simulink model "cos_sin_CORDIC"  (R2023b)
settings: Solver=FixedStepDiscrete  StartTime=0.0  StopTime=15*ts  RelTol=1e-3
undefined symbols (not defined in the file): ts
libraries: hdlsllib x30, simulink_extras x1
settings Model: DataTypeOverride=Off  Creator=adarwish  LastModifiedBy=hackathon_fpga
settings OptimizationCC: BlockReduction=off  ConditionallyExecuteInputs=off  DefaultParameterBehavior=Inlined  InheritOutputTypeSmallerThanSingle=on
settings DebuggingCC: AlgebraicLoopMsg=error  SingleTaskRateTransMsg=error  ParameterOverflowMsg=none  ParameterPrecisionLossMsg=none
settings HardwareCC: ProdBitPerPointer=32  ProdBitPerSizeT=32  ProdBitPerPtrDiffT=32  ProdLargestAtomicFloat=None  ProdIntDivRoundTo=Undefined  ProdEndianess=Unspecified  ProdWordSize=32  ProdHWDeviceType=ASIC/FPGA->ASIC/FPGA  TargetBitPerLong=64  TargetBitPerPointer=64  TargetBitPerSizeT=64  TargetBitPerPtrDiffT=64  TargetLongLongMode=on  TargetIntDivRoundTo=Zero  TargetEndianess=LittleEndian  TargetWordSize=64  TargetHWDeviceType=Custom Processor->MATLAB Host Computer  ProdEqTarget=off

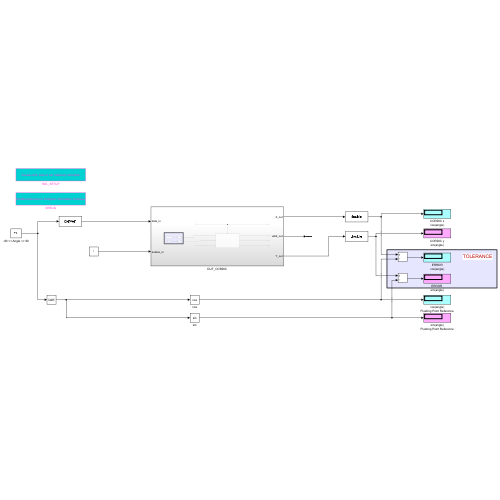
[thumbnail: Simulink's stored preview of the top-level diagram]
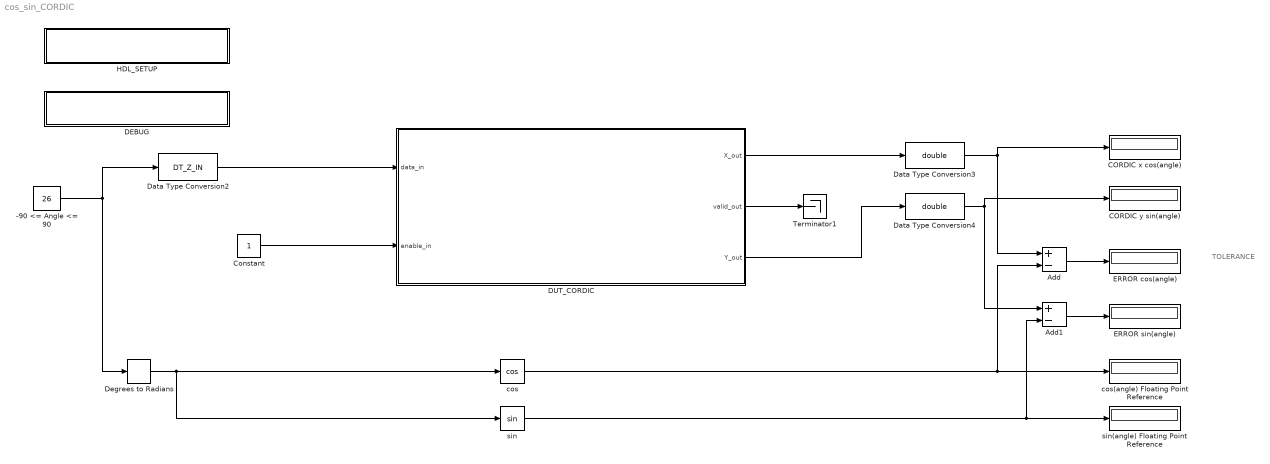
== system cos_sin_CORDIC ==
  note: TOLERANCE
  -90 <= Angle <= 90 : Constant  Value=26  SampleTime=ts
  Add : Sum  Inputs=+-
  Add1 : Sum  Inputs=+-
  CORDIC x cos(angle) : Display
  CORDIC y sin(angle) : Display
  Constant : Constant  OutDataTypeStr=boolean  SampleTime=-1
  DEBUG : Subsystem
      settings: OpenFcn=|
      | set_param(bdroot, 'ShowLineDimensions', 'on');
      | set_param(bdroot, 'SampleTimeColors', 'on');
      | set_param(bdroot, 'ShowLineDimensions', 'on');
      | disp('DONE Configuring Information Overlay')
      mask Display: disp(['Double-click here to configure Information Overlays'])
  DUT_CORDIC : Subsystem
  Data Type Conversion2 : DataTypeConversion  OutDataTypeStr=DT_Z_IN  RndMeth=Nearest  SampleTime=ts
  Data Type Conversion3 : DataTypeConversion  OutDataTypeStr=double  RndMeth=Nearest
  Data Type Conversion4 : DataTypeConversion  OutDataTypeStr=double  RndMeth=Nearest
  Degrees to Radians : simulink_extras/Transformations/Degrees to Radians
  ERROR cos(angle) : Display
  ERROR sin(angle) : Display
  HDL_SETUP : Subsystem
      settings: OpenFcn=hdlsetup(bdroot);
      mask Display: disp(['Double-click here to run hdlsetup command'])
  Terminator1 : Terminator
  cos : Trigonometry  Operator=cos
  cos(angle) Floating Point Reference : Display
  sin : Trigonometry
  sin(angle) Floating Point Reference : Display
  wires:
  sin/1 -> Add1/2, sin(angle) Floating Point Reference/1
  -90 <= Angle <= 90/1 -> Degrees to Radians/1, Data Type Conversion2/1
  Data Type Conversion4/1 -> CORDIC y sin(angle)/1, Add1/1
  Data Type Conversion3/1 -> CORDIC x cos(angle)/1, Add/1
  Add/1 -> ERROR cos(angle)/1
  Add1/1 -> ERROR sin(angle)/1
  Data Type Conversion2/1 -> DUT_CORDIC/1(data_in)
  cos/1 -> Add/2, cos(angle) Floating Point Reference/1
  Degrees to Radians/1 -> sin/1, cos/1
  Constant/1 -> DUT_CORDIC/2(enable_in)
  DUT_CORDIC/3(Y_out) -> Data Type Conversion4/1
  DUT_CORDIC/1(X_out) -> Data Type Conversion3/1
  DUT_CORDIC/2(valid_out) -> Terminator1/1

== system cos_sin_CORDIC/DEBUG ==

== system cos_sin_CORDIC/DUT_CORDIC ==
  note: PRE-SCALING
      | The input magnitude is prescaled to 1/1.6.
      | This means the finalmagnitude will be 1 and we do not need
      | to scale the output.
  data_in : Inport
  enable_in : Inport  Port=2
  1/Kn : Constant  Value=1/1.646743506596901  OutDataTypeStr=DT_X_IN  SampleTime=ts
  ALGORITHM : Subsystem
  Data Type Conversion : DataTypeConversion  OutDataTypeStr=DT_X_IN  RndMeth=Nearest  SampleTime=ts
  Data Type Conversion1 : DataTypeConversion  OutDataTypeStr=DT_Y_IN  RndMeth=Nearest  SampleTime=ts
  Set to 0 : Constant  Value=0  OutDataTypeStr=DT_Y_IN  SampleTime=ts
  Terminator : Terminator
  X_out : Outport
  valid_out : Outport  Port=2
  Y_out : Outport  Port=3
  wires:
  1/Kn/1 -> Data Type Conversion/1
  Set to 0/1 -> Data Type Conversion1/1
  Data Type Conversion/1 -> ALGORITHM/1(X In)
  Data Type Conversion1/1 -> ALGORITHM/2(Y In)
  data_in/1 -> ALGORITHM/3(Z In)
  ALGORITHM/3(Z Out) -> Terminator/1
  enable_in/1 -> ALGORITHM/Enable, valid_out/1
  ALGORITHM/1(X Out) -> X_out/1
  ALGORITHM/2(Y Out) -> Y_out/1

== system cos_sin_CORDIC/HDL_SETUP ==

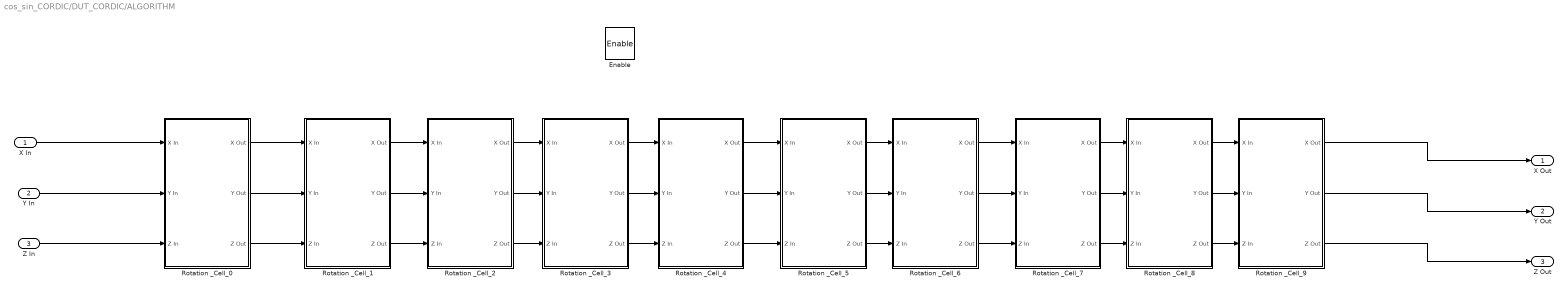
== system cos_sin_CORDIC/DUT_CORDIC/ALGORITHM ==
  X In : Inport
  Y In : Inport  Port=2
  Z In : Inport  Port=3
  Enable : EnablePort
  Rotation _Cell_0 : Subsystem  mask(Rotation Cell){i=0}
      mask prompts: i "Number of Iterations (i)"
  Rotation _Cell_1 : Subsystem  mask(Rotation Cell){i=1}
      mask prompts: i "Number of Iterations (i)"
  Rotation _Cell_2 : Subsystem  mask(Rotation Cell){i=2}
      mask prompts: i "Number of Iterations (i)"
  Rotation _Cell_3 : Subsystem  mask(Rotation Cell){i=3}
      mask prompts: i "Number of Iterations (i)"
  Rotation _Cell_4 : Subsystem  mask(Rotation Cell){i=4}
      mask prompts: i "Number of Iterations (i)"
  Rotation _Cell_5 : Subsystem  mask(Rotation Cell){i=5}
      mask prompts: i "Number of Iterations (i)"
  Rotation _Cell_6 : Subsystem  mask(Rotation Cell){i=6}
      mask prompts: i "Number of Iterations (i)"
  Rotation _Cell_7 : Subsystem  mask(Rotation Cell){i=7}
      mask prompts: i "Number of Iterations (i)"
  Rotation _Cell_8 : Subsystem  mask(Rotation Cell){i=8}
      mask prompts: i "Number of Iterations (i)"
  Rotation _Cell_9 : Subsystem  mask(Rotation Cell){i=9}
      mask prompts: i "Number of Iterations (i)"
  X Out : Outport  InitialOutput=0
  Y Out : Outport  Port=2  InitialOutput=0
  Z Out : Outport  Port=3  InitialOutput=0
  wires:
  Y In/1 -> Rotation _Cell_0/2(Y In)
  Rotation _Cell_0/2(Y Out) -> Rotation _Cell_1/2(Y In)
  Rotation _Cell_0/1(X Out) -> Rotation _Cell_1/1(X In)
  Rotation _Cell_0/3(Z Out) -> Rotation _Cell_1/3(Z In)
  X In/1 -> Rotation _Cell_0/1(X In)
  Z In/1 -> Rotation _Cell_0/3(Z In)
  Rotation _Cell_1/1(X Out) -> Rotation _Cell_2/1(X In)
  Rotation _Cell_1/2(Y Out) -> Rotation _Cell_2/2(Y In)
  Rotation _Cell_1/3(Z Out) -> Rotation _Cell_2/3(Z In)
  Rotation _Cell_2/1(X Out) -> Rotation _Cell_3/1(X In)
  Rotation _Cell_2/2(Y Out) -> Rotation _Cell_3/2(Y In)
  Rotation _Cell_2/3(Z Out) -> Rotation _Cell_3/3(Z In)
  Rotation _Cell_3/1(X Out) -> Rotation _Cell_4/1(X In)
  Rotation _Cell_3/2(Y Out) -> Rotation _Cell_4/2(Y In)
  Rotation _Cell_3/3(Z Out) -> Rotation _Cell_4/3(Z In)
  Rotation _Cell_4/1(X Out) -> Rotation _Cell_5/1(X In)
  Rotation _Cell_4/2(Y Out) -> Rotation _Cell_5/2(Y In)
  Rotation _Cell_4/3(Z Out) -> Rotation _Cell_5/3(Z In)
  Rotation _Cell_5/1(X Out) -> Rotation _Cell_6/1(X In)
  Rotation _Cell_5/2(Y Out) -> Rotation _Cell_6/2(Y In)
  Rotation _Cell_5/3(Z Out) -> Rotation _Cell_6/3(Z In)
  Rotation _Cell_6/1(X Out) -> Rotation _Cell_7/1(X In)
  Rotation _Cell_6/2(Y Out) -> Rotation _Cell_7/2(Y In)
  Rotation _Cell_6/3(Z Out) -> Rotation _Cell_7/3(Z In)
  Rotation _Cell_7/1(X Out) -> Rotation _Cell_8/1(X In)
  Rotation _Cell_7/2(Y Out) -> Rotation _Cell_8/2(Y In)
  Rotation _Cell_7/3(Z Out) -> Rotation _Cell_8/3(Z In)
  Rotation _Cell_8/1(X Out) -> Rotation _Cell_9/1(X In)
  Rotation _Cell_8/2(Y Out) -> Rotation _Cell_9/2(Y In)
  Rotation _Cell_8/3(Z Out) -> Rotation _Cell_9/3(Z In)
  Rotation _Cell_9/1(X Out) -> X Out/1
  Rotation _Cell_9/2(Y Out) -> Y Out/1
  Rotation _Cell_9/3(Z Out) -> Z Out/1

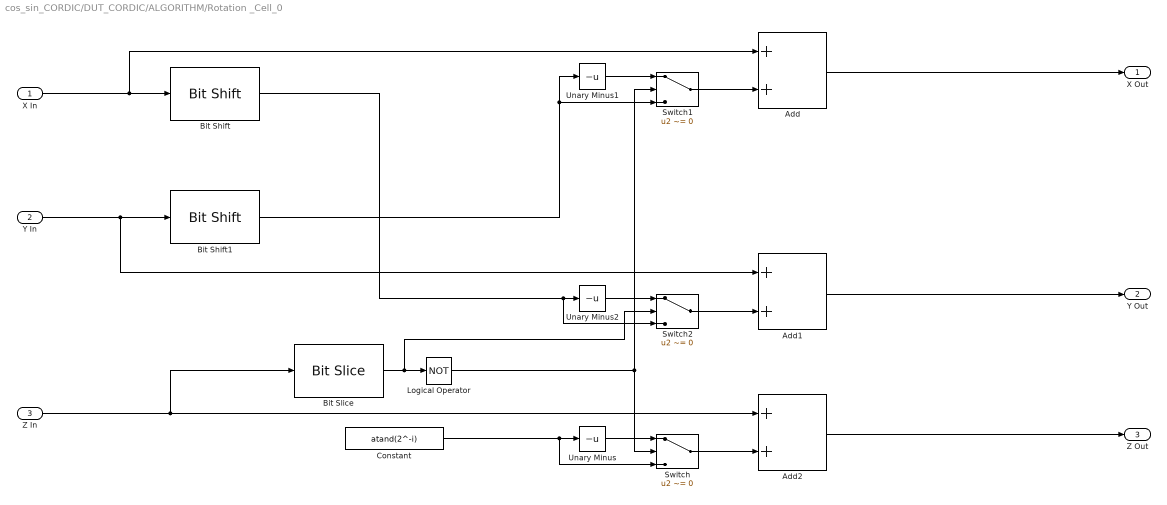
== system cos_sin_CORDIC/DUT_CORDIC/ALGORITHM/Rotation _Cell_0 ==
  X In : Inport
  Y In : Inport  Port=2
  Z In : Inport  Port=3
  Add : Sum  OutDataTypeStr=fixdt(1,15,12)
  Add1 : Sum  OutDataTypeStr=fixdt(1,15,12)
  Add2 : Sum  OutDataTypeStr=fixdt(1,20,12)
  Bit Shift : hdlsllib/Logic and Bit Operations/Bit Shift  mode=Shift Right Arithmetic  N=i
  Bit Shift1 : hdlsllib/Logic and Bit Operations/Bit Shift  mode=Shift Right Arithmetic  N=i
  Bit Slice : hdlsllib/Logic and Bit Operations/Bit Slice  lidx=19  ridx=19
  Constant : Constant  Value=atand(2^-i)  OutDataTypeStr=fixdt(1,20,12)  SampleTime=-1
  Logical Operator : Logic  Operator=NOT  AllPortsSameDT=off  OutDataTypeStr=boolean
  Switch : Switch  Criteria=u2 ~= 0  SaturateOnIntegerOverflow=off  InputSameDT=off
  Switch1 : Switch  Criteria=u2 ~= 0  SaturateOnIntegerOverflow=off  InputSameDT=off
  Switch2 : Switch  Criteria=u2 ~= 0  SaturateOnIntegerOverflow=off  InputSameDT=off
  Unary Minus : UnaryMinus
  Unary Minus1 : UnaryMinus
  Unary Minus2 : UnaryMinus
  X Out : Outport
  Y Out : Outport  Port=2
  Z Out : Outport  Port=3
  wires:
  Constant/1 -> Unary Minus/1, Switch/3
  Y In/1 -> Bit Shift1/1, Add1/1
  X In/1 -> Bit Shift/1, Add/1
  Add/1 -> X Out/1
  Unary Minus2/1 -> Switch2/1
  Unary Minus/1 -> Switch/1
  Add1/1 -> Y Out/1
  Switch1/1 -> Add/2
  Bit Shift/1 -> Switch2/3, Unary Minus2/1
  Switch2/1 -> Add1/2
  Unary Minus1/1 -> Switch1/1
  Bit Shift1/1 -> Switch1/3, Unary Minus1/1
  Z In/1 -> Bit Slice/1, Add2/1
  Bit Slice/1 -> Logical Operator/1, Switch2/2
  Switch/1 -> Add2/2
  Add2/1 -> Z Out/1
  Logical Operator/1 -> Switch/2, Switch1/2

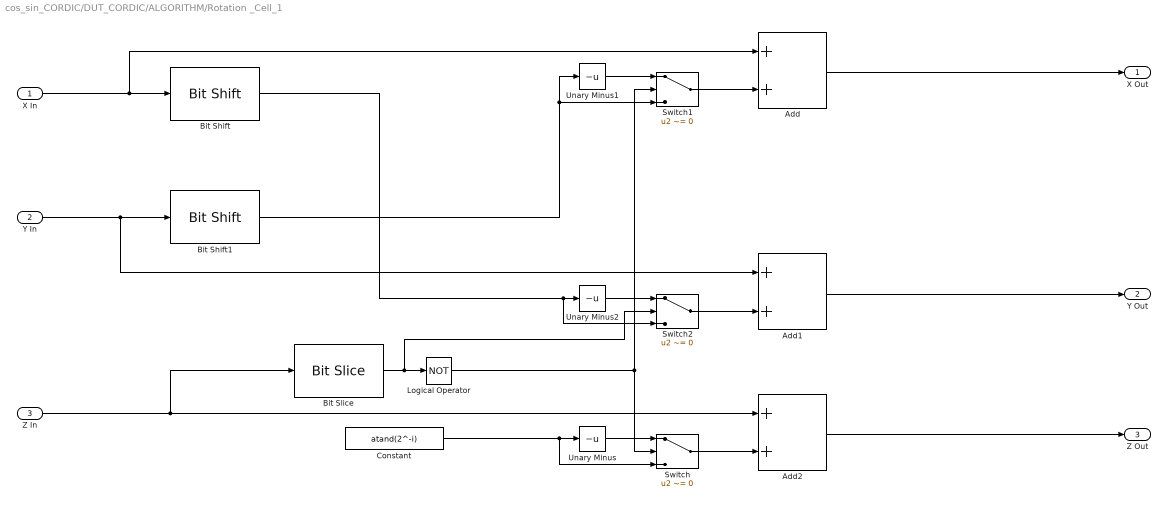
== system cos_sin_CORDIC/DUT_CORDIC/ALGORITHM/Rotation _Cell_1 ==
  X In : Inport
  Y In : Inport  Port=2
  Z In : Inport  Port=3
  Add : Sum  OutDataTypeStr=fixdt(1,15,12)
  Add1 : Sum  OutDataTypeStr=fixdt(1,15,12)
  Add2 : Sum  OutDataTypeStr=fixdt(1,20,12)
  Bit Shift : hdlsllib/Logic and Bit Operations/Bit Shift  mode=Shift Right Arithmetic  N=i
  Bit Shift1 : hdlsllib/Logic and Bit Operations/Bit Shift  mode=Shift Right Arithmetic  N=i
  Bit Slice : hdlsllib/Logic and Bit Operations/Bit Slice  lidx=19  ridx=19
  Constant : Constant  Value=atand(2^-i)  OutDataTypeStr=fixdt(1,20,12)  SampleTime=-1
  Logical Operator : Logic  Operator=NOT  AllPortsSameDT=off  OutDataTypeStr=boolean
  Switch : Switch  Criteria=u2 ~= 0  SaturateOnIntegerOverflow=off  InputSameDT=off
  Switch1 : Switch  Criteria=u2 ~= 0  SaturateOnIntegerOverflow=off  InputSameDT=off
  Switch2 : Switch  Criteria=u2 ~= 0  SaturateOnIntegerOverflow=off  InputSameDT=off
  Unary Minus : UnaryMinus
  Unary Minus1 : UnaryMinus
  Unary Minus2 : UnaryMinus
  X Out : Outport
  Y Out : Outport  Port=2
  Z Out : Outport  Port=3
  wires:
  Constant/1 -> Unary Minus/1, Switch/3
  Y In/1 -> Bit Shift1/1, Add1/1
  X In/1 -> Bit Shift/1, Add/1
  Add/1 -> X Out/1
  Unary Minus2/1 -> Switch2/1
  Unary Minus/1 -> Switch/1
  Add1/1 -> Y Out/1
  Switch1/1 -> Add/2
  Bit Shift/1 -> Switch2/3, Unary Minus2/1
  Switch2/1 -> Add1/2
  Unary Minus1/1 -> Switch1/1
  Bit Shift1/1 -> Switch1/3, Unary Minus1/1
  Z In/1 -> Bit Slice/1, Add2/1
  Bit Slice/1 -> Logical Operator/1, Switch2/2
  Switch/1 -> Add2/2
  Add2/1 -> Z Out/1
  Logical Operator/1 -> Switch/2, Switch1/2

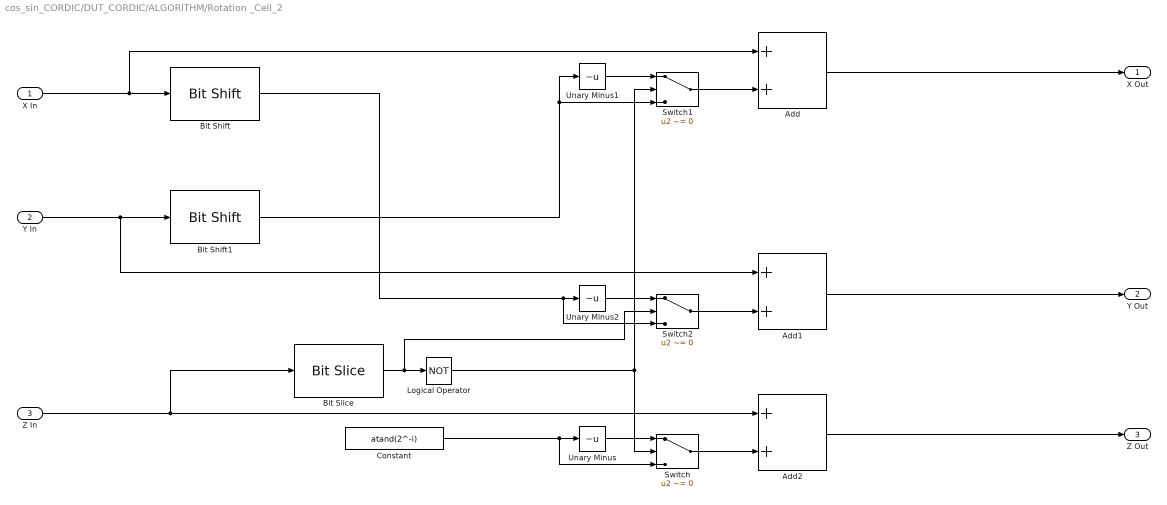
== system cos_sin_CORDIC/DUT_CORDIC/ALGORITHM/Rotation _Cell_2 ==
  X In : Inport
  Y In : Inport  Port=2
  Z In : Inport  Port=3
  Add : Sum  OutDataTypeStr=fixdt(1,15,12)
  Add1 : Sum  OutDataTypeStr=fixdt(1,15,12)
  Add2 : Sum  OutDataTypeStr=fixdt(1,20,12)
  Bit Shift : hdlsllib/Logic and Bit Operations/Bit Shift  mode=Shift Right Arithmetic  N=i
  Bit Shift1 : hdlsllib/Logic and Bit Operations/Bit Shift  mode=Shift Right Arithmetic  N=i
  Bit Slice : hdlsllib/Logic and Bit Operations/Bit Slice  lidx=19  ridx=19
  Constant : Constant  Value=atand(2^-i)  OutDataTypeStr=fixdt(1,20,12)  SampleTime=-1
  Logical Operator : Logic  Operator=NOT  AllPortsSameDT=off  OutDataTypeStr=boolean
  Switch : Switch  Criteria=u2 ~= 0  SaturateOnIntegerOverflow=off  InputSameDT=off
  Switch1 : Switch  Criteria=u2 ~= 0  SaturateOnIntegerOverflow=off  InputSameDT=off
  Switch2 : Switch  Criteria=u2 ~= 0  SaturateOnIntegerOverflow=off  InputSameDT=off
  Unary Minus : UnaryMinus
  Unary Minus1 : UnaryMinus
  Unary Minus2 : UnaryMinus
  X Out : Outport
  Y Out : Outport  Port=2
  Z Out : Outport  Port=3
  wires:
  Constant/1 -> Unary Minus/1, Switch/3
  Y In/1 -> Bit Shift1/1, Add1/1
  X In/1 -> Bit Shift/1, Add/1
  Add/1 -> X Out/1
  Unary Minus2/1 -> Switch2/1
  Unary Minus/1 -> Switch/1
  Add1/1 -> Y Out/1
  Switch1/1 -> Add/2
  Bit Shift/1 -> Switch2/3, Unary Minus2/1
  Switch2/1 -> Add1/2
  Unary Minus1/1 -> Switch1/1
  Bit Shift1/1 -> Switch1/3, Unary Minus1/1
  Z In/1 -> Bit Slice/1, Add2/1
  Bit Slice/1 -> Logical Operator/1, Switch2/2
  Switch/1 -> Add2/2
  Add2/1 -> Z Out/1
  Logical Operator/1 -> Switch/2, Switch1/2

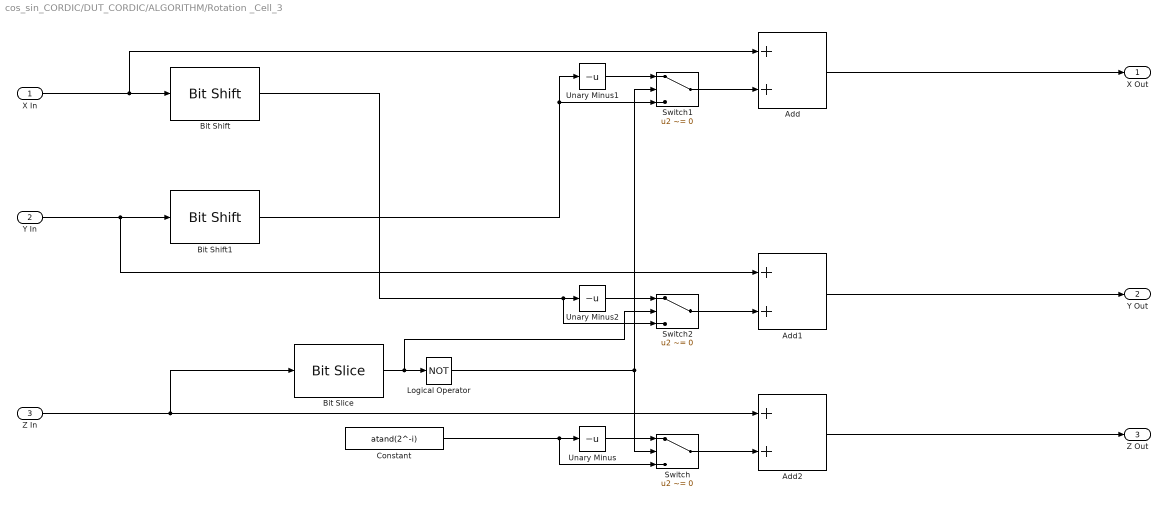
== system cos_sin_CORDIC/DUT_CORDIC/ALGORITHM/Rotation _Cell_3 ==
  X In : Inport
  Y In : Inport  Port=2
  Z In : Inport  Port=3
  Add : Sum  OutDataTypeStr=fixdt(1,15,12)
  Add1 : Sum  OutDataTypeStr=fixdt(1,15,12)
  Add2 : Sum  OutDataTypeStr=fixdt(1,20,12)
  Bit Shift : hdlsllib/Logic and Bit Operations/Bit Shift  mode=Shift Right Arithmetic  N=i
  Bit Shift1 : hdlsllib/Logic and Bit Operations/Bit Shift  mode=Shift Right Arithmetic  N=i
  Bit Slice : hdlsllib/Logic and Bit Operations/Bit Slice  lidx=19  ridx=19
  Constant : Constant  Value=atand(2^-i)  OutDataTypeStr=fixdt(1,20,12)  SampleTime=-1
  Logical Operator : Logic  Operator=NOT  AllPortsSameDT=off  OutDataTypeStr=boolean
  Switch : Switch  Criteria=u2 ~= 0  SaturateOnIntegerOverflow=off  InputSameDT=off
  Switch1 : Switch  Criteria=u2 ~= 0  SaturateOnIntegerOverflow=off  InputSameDT=off
  Switch2 : Switch  Criteria=u2 ~= 0  SaturateOnIntegerOverflow=off  InputSameDT=off
  Unary Minus : UnaryMinus
  Unary Minus1 : UnaryMinus
  Unary Minus2 : UnaryMinus
  X Out : Outport
  Y Out : Outport  Port=2
  Z Out : Outport  Port=3
  wires:
  Constant/1 -> Unary Minus/1, Switch/3
  Y In/1 -> Bit Shift1/1, Add1/1
  X In/1 -> Bit Shift/1, Add/1
  Add/1 -> X Out/1
  Unary Minus2/1 -> Switch2/1
  Unary Minus/1 -> Switch/1
  Add1/1 -> Y Out/1
  Switch1/1 -> Add/2
  Bit Shift/1 -> Switch2/3, Unary Minus2/1
  Switch2/1 -> Add1/2
  Unary Minus1/1 -> Switch1/1
  Bit Shift1/1 -> Switch1/3, Unary Minus1/1
  Z In/1 -> Bit Slice/1, Add2/1
  Bit Slice/1 -> Logical Operator/1, Switch2/2
  Switch/1 -> Add2/2
  Add2/1 -> Z Out/1
  Logical Operator/1 -> Switch/2, Switch1/2

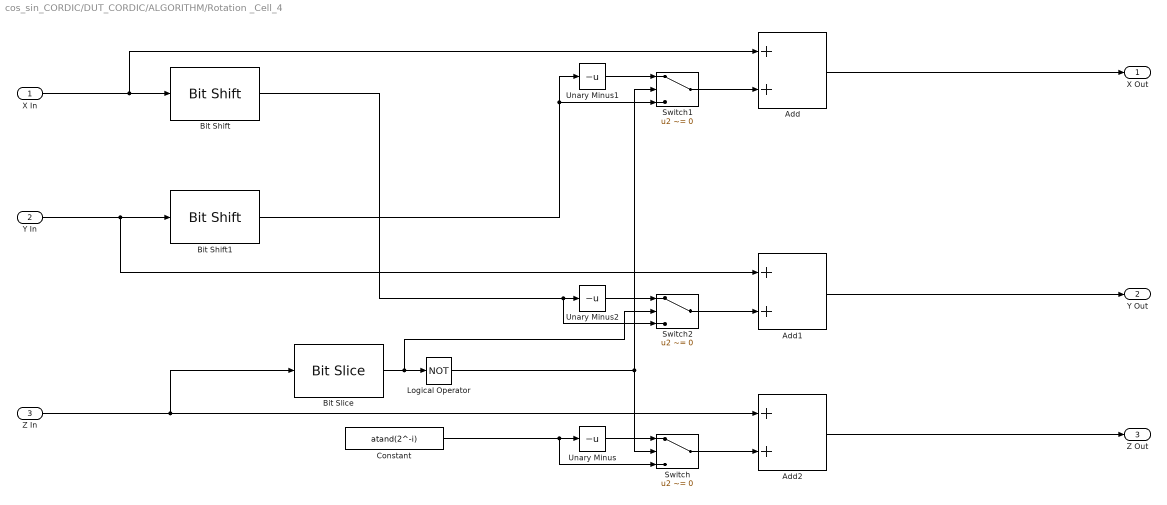
== system cos_sin_CORDIC/DUT_CORDIC/ALGORITHM/Rotation _Cell_4 ==
  X In : Inport
  Y In : Inport  Port=2
  Z In : Inport  Port=3
  Add : Sum  OutDataTypeStr=fixdt(1,15,12)
  Add1 : Sum  OutDataTypeStr=fixdt(1,15,12)
  Add2 : Sum  OutDataTypeStr=fixdt(1,20,12)
  Bit Shift : hdlsllib/Logic and Bit Operations/Bit Shift  mode=Shift Right Arithmetic  N=i
  Bit Shift1 : hdlsllib/Logic and Bit Operations/Bit Shift  mode=Shift Right Arithmetic  N=i
  Bit Slice : hdlsllib/Logic and Bit Operations/Bit Slice  lidx=19  ridx=19
  Constant : Constant  Value=atand(2^-i)  OutDataTypeStr=fixdt(1,20,12)  SampleTime=-1
  Logical Operator : Logic  Operator=NOT  AllPortsSameDT=off  OutDataTypeStr=boolean
  Switch : Switch  Criteria=u2 ~= 0  SaturateOnIntegerOverflow=off  InputSameDT=off
  Switch1 : Switch  Criteria=u2 ~= 0  SaturateOnIntegerOverflow=off  InputSameDT=off
  Switch2 : Switch  Criteria=u2 ~= 0  SaturateOnIntegerOverflow=off  InputSameDT=off
  Unary Minus : UnaryMinus
  Unary Minus1 : UnaryMinus
  Unary Minus2 : UnaryMinus
  X Out : Outport
  Y Out : Outport  Port=2
  Z Out : Outport  Port=3
  wires:
  Constant/1 -> Unary Minus/1, Switch/3
  Y In/1 -> Bit Shift1/1, Add1/1
  X In/1 -> Bit Shift/1, Add/1
  Add/1 -> X Out/1
  Unary Minus2/1 -> Switch2/1
  Unary Minus/1 -> Switch/1
  Add1/1 -> Y Out/1
  Switch1/1 -> Add/2
  Bit Shift/1 -> Switch2/3, Unary Minus2/1
  Switch2/1 -> Add1/2
  Unary Minus1/1 -> Switch1/1
  Bit Shift1/1 -> Switch1/3, Unary Minus1/1
  Z In/1 -> Bit Slice/1, Add2/1
  Bit Slice/1 -> Logical Operator/1, Switch2/2
  Switch/1 -> Add2/2
  Add2/1 -> Z Out/1
  Logical Operator/1 -> Switch/2, Switch1/2

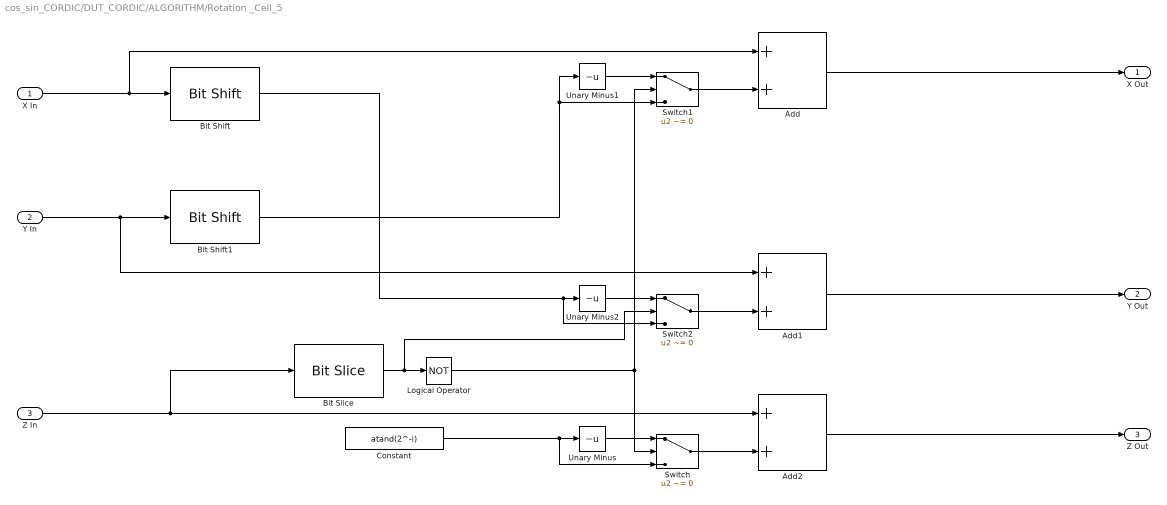
== system cos_sin_CORDIC/DUT_CORDIC/ALGORITHM/Rotation _Cell_5 ==
  X In : Inport
  Y In : Inport  Port=2
  Z In : Inport  Port=3
  Add : Sum  OutDataTypeStr=fixdt(1,15,12)
  Add1 : Sum  OutDataTypeStr=fixdt(1,15,12)
  Add2 : Sum  OutDataTypeStr=fixdt(1,20,12)
  Bit Shift : hdlsllib/Logic and Bit Operations/Bit Shift  mode=Shift Right Arithmetic  N=i
  Bit Shift1 : hdlsllib/Logic and Bit Operations/Bit Shift  mode=Shift Right Arithmetic  N=i
  Bit Slice : hdlsllib/Logic and Bit Operations/Bit Slice  lidx=19  ridx=19
  Constant : Constant  Value=atand(2^-i)  OutDataTypeStr=fixdt(1,20,12)  SampleTime=-1
  Logical Operator : Logic  Operator=NOT  AllPortsSameDT=off  OutDataTypeStr=boolean
  Switch : Switch  Criteria=u2 ~= 0  SaturateOnIntegerOverflow=off  InputSameDT=off
  Switch1 : Switch  Criteria=u2 ~= 0  SaturateOnIntegerOverflow=off  InputSameDT=off
  Switch2 : Switch  Criteria=u2 ~= 0  SaturateOnIntegerOverflow=off  InputSameDT=off
  Unary Minus : UnaryMinus
  Unary Minus1 : UnaryMinus
  Unary Minus2 : UnaryMinus
  X Out : Outport
  Y Out : Outport  Port=2
  Z Out : Outport  Port=3
  wires:
  Constant/1 -> Unary Minus/1, Switch/3
  Y In/1 -> Bit Shift1/1, Add1/1
  X In/1 -> Bit Shift/1, Add/1
  Add/1 -> X Out/1
  Unary Minus2/1 -> Switch2/1
  Unary Minus/1 -> Switch/1
  Add1/1 -> Y Out/1
  Switch1/1 -> Add/2
  Bit Shift/1 -> Switch2/3, Unary Minus2/1
  Switch2/1 -> Add1/2
  Unary Minus1/1 -> Switch1/1
  Bit Shift1/1 -> Switch1/3, Unary Minus1/1
  Z In/1 -> Bit Slice/1, Add2/1
  Bit Slice/1 -> Logical Operator/1, Switch2/2
  Switch/1 -> Add2/2
  Add2/1 -> Z Out/1
  Logical Operator/1 -> Switch/2, Switch1/2

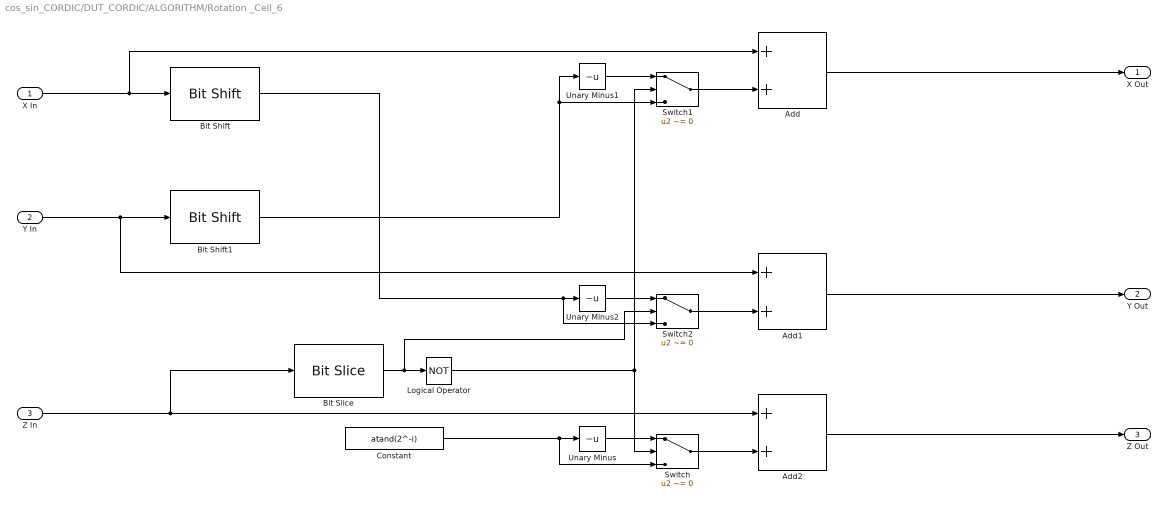
== system cos_sin_CORDIC/DUT_CORDIC/ALGORITHM/Rotation _Cell_6 ==
  X In : Inport
  Y In : Inport  Port=2
  Z In : Inport  Port=3
  Add : Sum  OutDataTypeStr=fixdt(1,15,12)
  Add1 : Sum  OutDataTypeStr=fixdt(1,15,12)
  Add2 : Sum  OutDataTypeStr=fixdt(1,20,12)
  Bit Shift : hdlsllib/Logic and Bit Operations/Bit Shift  mode=Shift Right Arithmetic  N=i
  Bit Shift1 : hdlsllib/Logic and Bit Operations/Bit Shift  mode=Shift Right Arithmetic  N=i
  Bit Slice : hdlsllib/Logic and Bit Operations/Bit Slice  lidx=19  ridx=19
  Constant : Constant  Value=atand(2^-i)  OutDataTypeStr=fixdt(1,20,12)  SampleTime=-1
  Logical Operator : Logic  Operator=NOT  AllPortsSameDT=off  OutDataTypeStr=boolean
  Switch : Switch  Criteria=u2 ~= 0  SaturateOnIntegerOverflow=off  InputSameDT=off
  Switch1 : Switch  Criteria=u2 ~= 0  SaturateOnIntegerOverflow=off  InputSameDT=off
  Switch2 : Switch  Criteria=u2 ~= 0  SaturateOnIntegerOverflow=off  InputSameDT=off
  Unary Minus : UnaryMinus
  Unary Minus1 : UnaryMinus
  Unary Minus2 : UnaryMinus
  X Out : Outport
  Y Out : Outport  Port=2
  Z Out : Outport  Port=3
  wires:
  Constant/1 -> Unary Minus/1, Switch/3
  Y In/1 -> Bit Shift1/1, Add1/1
  X In/1 -> Bit Shift/1, Add/1
  Add/1 -> X Out/1
  Unary Minus2/1 -> Switch2/1
  Unary Minus/1 -> Switch/1
  Add1/1 -> Y Out/1
  Switch1/1 -> Add/2
  Bit Shift/1 -> Switch2/3, Unary Minus2/1
  Switch2/1 -> Add1/2
  Unary Minus1/1 -> Switch1/1
  Bit Shift1/1 -> Switch1/3, Unary Minus1/1
  Z In/1 -> Bit Slice/1, Add2/1
  Bit Slice/1 -> Logical Operator/1, Switch2/2
  Switch/1 -> Add2/2
  Add2/1 -> Z Out/1
  Logical Operator/1 -> Switch/2, Switch1/2

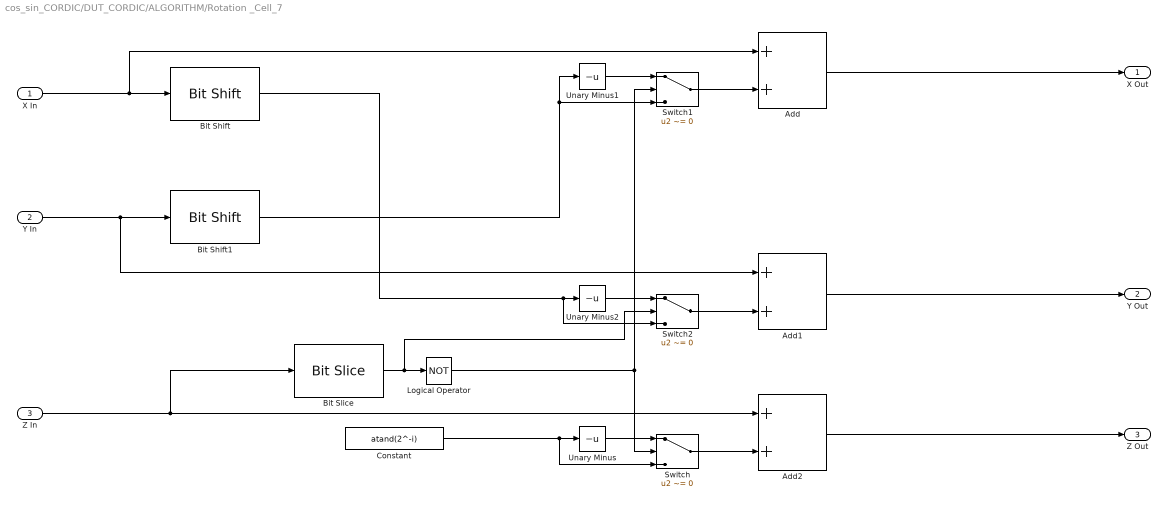
== system cos_sin_CORDIC/DUT_CORDIC/ALGORITHM/Rotation _Cell_7 ==
  X In : Inport
  Y In : Inport  Port=2
  Z In : Inport  Port=3
  Add : Sum  OutDataTypeStr=fixdt(1,15,12)
  Add1 : Sum  OutDataTypeStr=fixdt(1,15,12)
  Add2 : Sum  OutDataTypeStr=fixdt(1,20,12)
  Bit Shift : hdlsllib/Logic and Bit Operations/Bit Shift  mode=Shift Right Arithmetic  N=i
  Bit Shift1 : hdlsllib/Logic and Bit Operations/Bit Shift  mode=Shift Right Arithmetic  N=i
  Bit Slice : hdlsllib/Logic and Bit Operations/Bit Slice  lidx=19  ridx=19
  Constant : Constant  Value=atand(2^-i)  OutDataTypeStr=fixdt(1,20,12)  SampleTime=-1
  Logical Operator : Logic  Operator=NOT  AllPortsSameDT=off  OutDataTypeStr=boolean
  Switch : Switch  Criteria=u2 ~= 0  SaturateOnIntegerOverflow=off  InputSameDT=off
  Switch1 : Switch  Criteria=u2 ~= 0  SaturateOnIntegerOverflow=off  InputSameDT=off
  Switch2 : Switch  Criteria=u2 ~= 0  SaturateOnIntegerOverflow=off  InputSameDT=off
  Unary Minus : UnaryMinus
  Unary Minus1 : UnaryMinus
  Unary Minus2 : UnaryMinus
  X Out : Outport
  Y Out : Outport  Port=2
  Z Out : Outport  Port=3
  wires:
  Constant/1 -> Unary Minus/1, Switch/3
  Y In/1 -> Bit Shift1/1, Add1/1
  X In/1 -> Bit Shift/1, Add/1
  Add/1 -> X Out/1
  Unary Minus2/1 -> Switch2/1
  Unary Minus/1 -> Switch/1
  Add1/1 -> Y Out/1
  Switch1/1 -> Add/2
  Bit Shift/1 -> Switch2/3, Unary Minus2/1
  Switch2/1 -> Add1/2
  Unary Minus1/1 -> Switch1/1
  Bit Shift1/1 -> Switch1/3, Unary Minus1/1
  Z In/1 -> Bit Slice/1, Add2/1
  Bit Slice/1 -> Logical Operator/1, Switch2/2
  Switch/1 -> Add2/2
  Add2/1 -> Z Out/1
  Logical Operator/1 -> Switch/2, Switch1/2

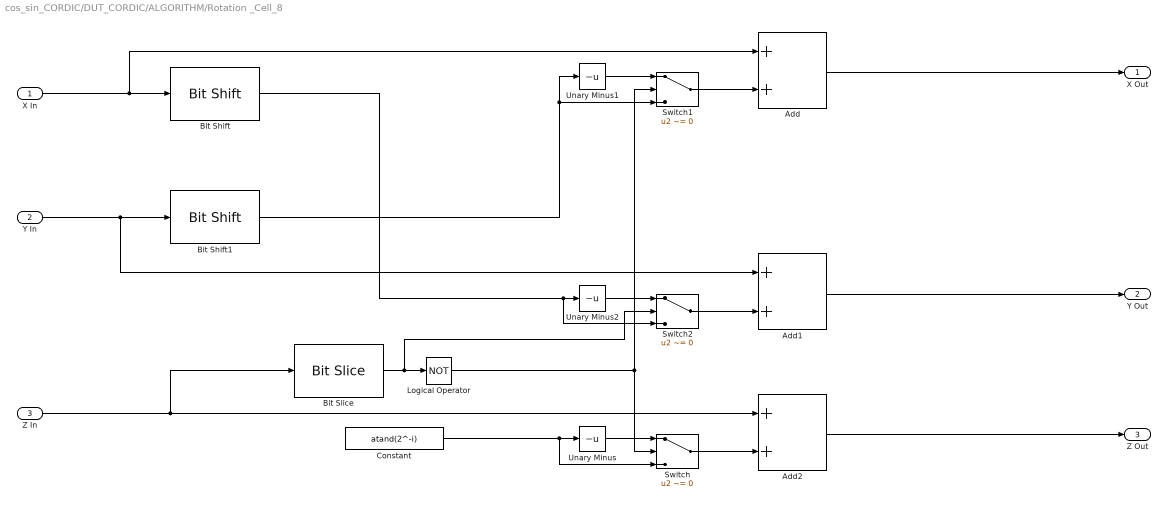
== system cos_sin_CORDIC/DUT_CORDIC/ALGORITHM/Rotation _Cell_8 ==
  X In : Inport
  Y In : Inport  Port=2
  Z In : Inport  Port=3
  Add : Sum  OutDataTypeStr=fixdt(1,15,12)
  Add1 : Sum  OutDataTypeStr=fixdt(1,15,12)
  Add2 : Sum  OutDataTypeStr=fixdt(1,20,12)
  Bit Shift : hdlsllib/Logic and Bit Operations/Bit Shift  mode=Shift Right Arithmetic  N=i
  Bit Shift1 : hdlsllib/Logic and Bit Operations/Bit Shift  mode=Shift Right Arithmetic  N=i
  Bit Slice : hdlsllib/Logic and Bit Operations/Bit Slice  lidx=19  ridx=19
  Constant : Constant  Value=atand(2^-i)  OutDataTypeStr=fixdt(1,20,12)  SampleTime=-1
  Logical Operator : Logic  Operator=NOT  AllPortsSameDT=off  OutDataTypeStr=boolean
  Switch : Switch  Criteria=u2 ~= 0  SaturateOnIntegerOverflow=off  InputSameDT=off
  Switch1 : Switch  Criteria=u2 ~= 0  SaturateOnIntegerOverflow=off  InputSameDT=off
  Switch2 : Switch  Criteria=u2 ~= 0  SaturateOnIntegerOverflow=off  InputSameDT=off
  Unary Minus : UnaryMinus
  Unary Minus1 : UnaryMinus
  Unary Minus2 : UnaryMinus
  X Out : Outport
  Y Out : Outport  Port=2
  Z Out : Outport  Port=3
  wires:
  Constant/1 -> Unary Minus/1, Switch/3
  Y In/1 -> Bit Shift1/1, Add1/1
  X In/1 -> Bit Shift/1, Add/1
  Add/1 -> X Out/1
  Unary Minus2/1 -> Switch2/1
  Unary Minus/1 -> Switch/1
  Add1/1 -> Y Out/1
  Switch1/1 -> Add/2
  Bit Shift/1 -> Switch2/3, Unary Minus2/1
  Switch2/1 -> Add1/2
  Unary Minus1/1 -> Switch1/1
  Bit Shift1/1 -> Switch1/3, Unary Minus1/1
  Z In/1 -> Bit Slice/1, Add2/1
  Bit Slice/1 -> Logical Operator/1, Switch2/2
  Switch/1 -> Add2/2
  Add2/1 -> Z Out/1
  Logical Operator/1 -> Switch/2, Switch1/2

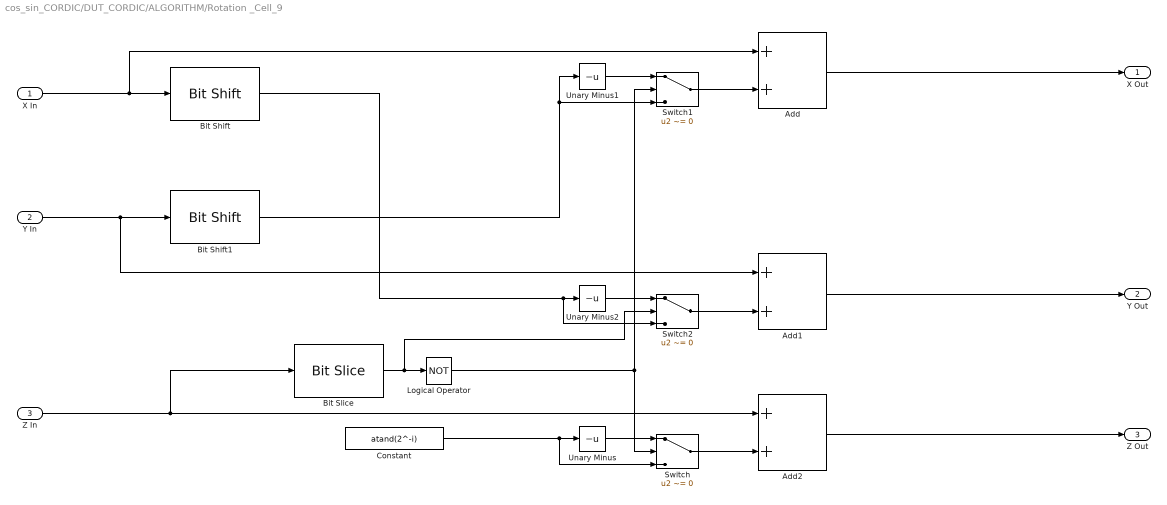
== system cos_sin_CORDIC/DUT_CORDIC/ALGORITHM/Rotation _Cell_9 ==
  X In : Inport
  Y In : Inport  Port=2
  Z In : Inport  Port=3
  Add : Sum  OutDataTypeStr=fixdt(1,15,12)
  Add1 : Sum  OutDataTypeStr=fixdt(1,15,12)
  Add2 : Sum  OutDataTypeStr=fixdt(1,20,12)
  Bit Shift : hdlsllib/Logic and Bit Operations/Bit Shift  mode=Shift Right Arithmetic  N=i
  Bit Shift1 : hdlsllib/Logic and Bit Operations/Bit Shift  mode=Shift Right Arithmetic  N=i
  Bit Slice : hdlsllib/Logic and Bit Operations/Bit Slice  lidx=19  ridx=19
  Constant : Constant  Value=atand(2^-i)  OutDataTypeStr=fixdt(1,20,12)  SampleTime=-1
  Logical Operator : Logic  Operator=NOT  AllPortsSameDT=off  OutDataTypeStr=boolean
  Switch : Switch  Criteria=u2 ~= 0  SaturateOnIntegerOverflow=off  InputSameDT=off
  Switch1 : Switch  Criteria=u2 ~= 0  SaturateOnIntegerOverflow=off  InputSameDT=off
  Switch2 : Switch  Criteria=u2 ~= 0  SaturateOnIntegerOverflow=off  InputSameDT=off
  Unary Minus : UnaryMinus
  Unary Minus1 : UnaryMinus
  Unary Minus2 : UnaryMinus
  X Out : Outport
  Y Out : Outport  Port=2
  Z Out : Outport  Port=3
  wires:
  Constant/1 -> Unary Minus/1, Switch/3
  Y In/1 -> Bit Shift1/1, Add1/1
  X In/1 -> Bit Shift/1, Add/1
  Add/1 -> X Out/1
  Unary Minus2/1 -> Switch2/1
  Unary Minus/1 -> Switch/1
  Add1/1 -> Y Out/1
  Switch1/1 -> Add/2
  Bit Shift/1 -> Switch2/3, Unary Minus2/1
  Switch2/1 -> Add1/2
  Unary Minus1/1 -> Switch1/1
  Bit Shift1/1 -> Switch1/3, Unary Minus1/1
  Z In/1 -> Bit Slice/1, Add2/1
  Bit Slice/1 -> Logical Operator/1, Switch2/2
  Switch/1 -> Add2/2
  Add2/1 -> Z Out/1
  Logical Operator/1 -> Switch/2, Switch1/2
